simulink model "ClosedLoopBallandBeam"  (R2019a)
settings: Solver=ode4  StartTime=0.0  StopTime=10.0  FixedStep=0.005  RelTol=1e-3
values from neighbouring files (symbols this model uses):
  a1 = -(Km*Ke)/(J*Rm)    [BallandBeamModeling.m]
  a2 = -(wball)/J    (= -33.5116157375)    [BallandBeamModeling.m]
  a3 = (5*g)/7    (= 7.00714285714)    [BallandBeamModeling.m]
  b1 = Km/(J*Rm)    [BallandBeamModeling.m]
  initTheta = 30/180*pi    (= 0.523598775598)    [BallandBeamModeling.m]
  initX = 0.00    (= 0)    [BallandBeamModeling.m]
  K = acker(A,B,poles)    [BallandBeamModeling.m]
settings Model: Creator=xde12  LastModifiedBy=xde12

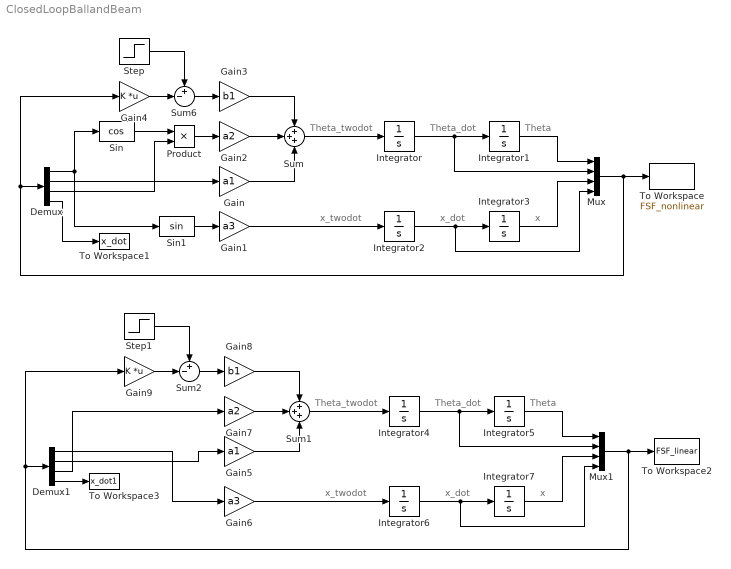
== system ClosedLoopBallandBeam ==
  note: Theta
  note: Theta_dot
  note: x_dot
  note: x
  note: Theta_twodot
  note: x_twodot
  note: Theta
  note: Theta_dot
  note: x_twodot
  note: x
  note: Theta_twodot
  note: x_dot
  Demux : Demux
  Demux1 : Demux
  Gain : Gain  Gain=a1
  Gain1 : Gain  Gain=a3
  Gain2 : Gain  Gain=a2
  Gain3 : Gain  Gain=b1
  Gain4 : Gain  Gain=K  Multiplication=Matrix(K*u)
  Gain5 : Gain  Gain=a1
  Gain6 : Gain  Gain=a3
  Gain7 : Gain  Gain=a2
  Gain8 : Gain  Gain=b1
  Gain9 : Gain  Gain=K  Multiplication=Matrix(K*u)
  Integrator{,2,4,6} (4 alike) : Integrator
  Integrator1 : Integrator  InitialCondition=initTheta
  Integrator3 : Integrator  InitialCondition=initX
  Integrator5 : Integrator  InitialCondition=initTheta
  Integrator7 : Integrator  InitialCondition=initX
  Mux : Mux
  Mux1 : Mux
  Product : Product
  Sin : Trigonometry  Operator=cos
  Sin1 : Trigonometry
  Step : Step  After=0  SampleTime=0.005
  Step1 : Step  After=0  SampleTime=0.005
  Sum : Sum  Inputs=+++
  Sum1 : Sum  Inputs=+++
  Sum2 : Sum  Inputs=+-|
  Sum6 : Sum  Inputs=+-|
  To Workspace : ToWorkspace  VariableName=FSF_nonlinear  SaveFormat=Structure With Time  SampleTime=0.005
  To Workspace1 : ToWorkspace  VariableName=x_dot  SaveFormat=Structure With Time  SampleTime=0.005
  To Workspace2 : ToWorkspace  VariableName=FSF_linear  SaveFormat=Structure With Time  SampleTime=0.005
  To Workspace3 : ToWorkspace  VariableName=x_dot1  SaveFormat=Structure With Time  SampleTime=0.005
  wires:
  Integrator/1 -> Mux/2, Integrator1/1
  Integrator2/1 -> Mux/4, Integrator3/1
  Mux/1 -> To Workspace/1, Gain4/1, Demux/1
  Product/1 -> Gain2/1
  Sum/1 -> Integrator/1
  Gain1/1 -> Integrator2/1
  Sin/1 -> Product/1
  Gain3/1 -> Sum/1
  Integrator3/1 -> Mux/3
  Demux/3 -> Product/2
  Gain4/1 -> Sum6/2
  Sum6/1 -> Gain3/1
  Integrator1/1 -> Mux/1
  Gain2/1 -> Sum/2
  Step/1 -> Sum6/1
  Demux/4 -> To Workspace1/1
  Sin1/1 -> Gain1/1
  Demux/1 -> Sin/1, Sin1/1
  Demux/2 -> Gain/1
  Gain/1 -> Sum/3
  Integrator5/1 -> Mux1/1
  Demux1/1 -> Gain6/1
  Demux1/2 -> Gain5/1
  Mux1/1 -> To Workspace2/1, Gain9/1, Demux1/1
  Gain9/1 -> Sum2/2
  Step1/1 -> Sum2/1
  Sum2/1 -> Gain8/1
  Demux1/4 -> To Workspace3/1
  Gain5/1 -> Sum1/3
  Sum1/1 -> Integrator4/1
  Demux1/3 -> Gain7/1
  Integrator7/1 -> Mux1/3
  Gain7/1 -> Sum1/2
  Integrator4/1 -> Mux1/2, Integrator5/1
  Integrator6/1 -> Mux1/4, Integrator7/1
  Gain8/1 -> Sum1/1
  Gain6/1 -> Integrator6/1
